simulink library "dragTurbine"  (R2020a)
settings: Solver=VariableStepAuto  StartTime=0.0  StopTime=10.0  RelTol=1e-3
undefined symbols (not defined in the file): alph, eta1, rho, tsrTab, vcl
libraries: simulink x3, vrlib x2, alphaBeta_ul x1, localApparentWind_ul x1
settings Model: Creator=Ayaz  LastModifiedBy=adabney
settings DataIOCC: ReturnWorkspaceOutputs=off
settings DebuggingCC: ArithmeticOperatorsInVariantConditions=warning
settings SFSimCC: CustomCodeUndefinedFunction=UseInterfaceOnly

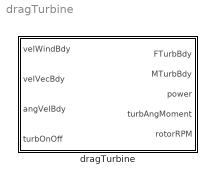
== system dragTurbine ==
  dragTurbine : Subsystem  TreatAsAtomicUnit=on  mask{vhcl=vcl}
      mask prompts: vhcl "Vehicle Object"

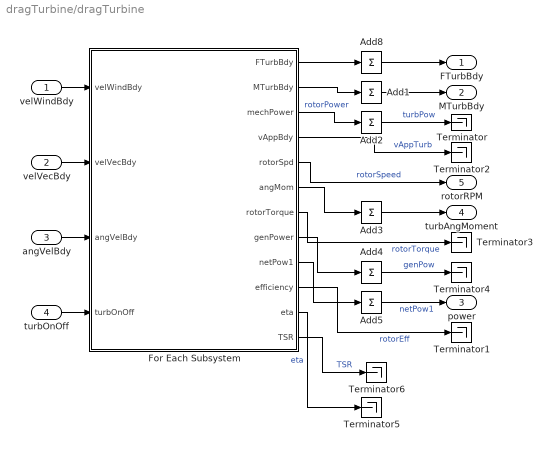
== system dragTurbine/dragTurbine ==
  velWindBdy : Inport
  velVecBdy : Inport  Port=2
  angVelBdy : Inport  Port=3
  turbOnOff : Inport  Port=4
  Add{1..3,8} (4 alike) : Sum  Inputs=1  CollapseMode=Specified dimension  CollapseDim=2
  Add4 : Sum  Inputs=1  CollapseDim=2
  Add5 : Sum  Inputs=1  CollapseDim=2
  For Each Subsystem : Subsystem  TreatAsAtomicUnit=on  mask{rho=rho, turb_struct=vhcl.struct('OCT.turb'), vhcl=vhcl}
      mask prompts: rho "Fluid Density"; turb_struct "Turbine Structure"; vhcl "Vehicle"
  Terminator{,1..6} (7 alike) : Terminator
  FTurbBdy : Outport  PortDimensions=[3,1]  VectorParamsAs1DForOutWhenUnconnected=off
  MTurbBdy : Outport  Port=2  PortDimensions=[3,1]  VectorParamsAs1DForOutWhenUnconnected=off
  power : Outport  Port=3  PortDimensions=[1,1]  VectorParamsAs1DForOutWhenUnconnected=off
  turbAngMoment : Outport  Port=4  PortDimensions=[3,1]  VectorParamsAs1DForOutWhenUnconnected=off
  rotorRPM : Outport  Port=5  VectorParamsAs1DForOutWhenUnconnected=off
  wires:
  velVecBdy/1 -> For Each Subsystem/2(velVecBdy)
  angVelBdy/1 -> For Each Subsystem/3(angVelBdy)
  turbOnOff/1 -> For Each Subsystem/4(turbOnOff)
  For Each Subsystem/1(FTurbBdy) -> Add8/1
  For Each Subsystem/2(MTurbBdy) -> Add1/1
  velWindBdy/1 -> For Each Subsystem/1(velWindBdy)
  Add8/1 -> FTurbBdy/1
  Add1/1 -> MTurbBdy/1
  For Each Subsystem/5(rotorSpd) -> rotorRPM/1  "rotorSpeed"
  For Each Subsystem/3(mechPower) -> Add2/1  "rotorPower"
  Add2/1 -> Terminator/1  "turbPow"
  For Each Subsystem/6(angMom) -> Add3/1
  Add3/1 -> turbAngMoment/1
  For Each Subsystem/4(vAppBdy) -> Terminator2/1  "vAppTurb"
  For Each Subsystem/7(rotorTorque) -> Terminator3/1  "rotorTorque"
  For Each Subsystem/8(genPower) -> Add4/1
  Add4/1 -> Terminator4/1  "genPow"
  For Each Subsystem/10(efficiency) -> Terminator1/1  "rotorEff"
  For Each Subsystem/9(netPow1) -> Add5/1
  Add5/1 -> power/1  "netPow1"
  For Each Subsystem/11(eta) -> Terminator5/1  "eta"
  For Each Subsystem/12(TSR) -> Terminator6/1  "TSR"

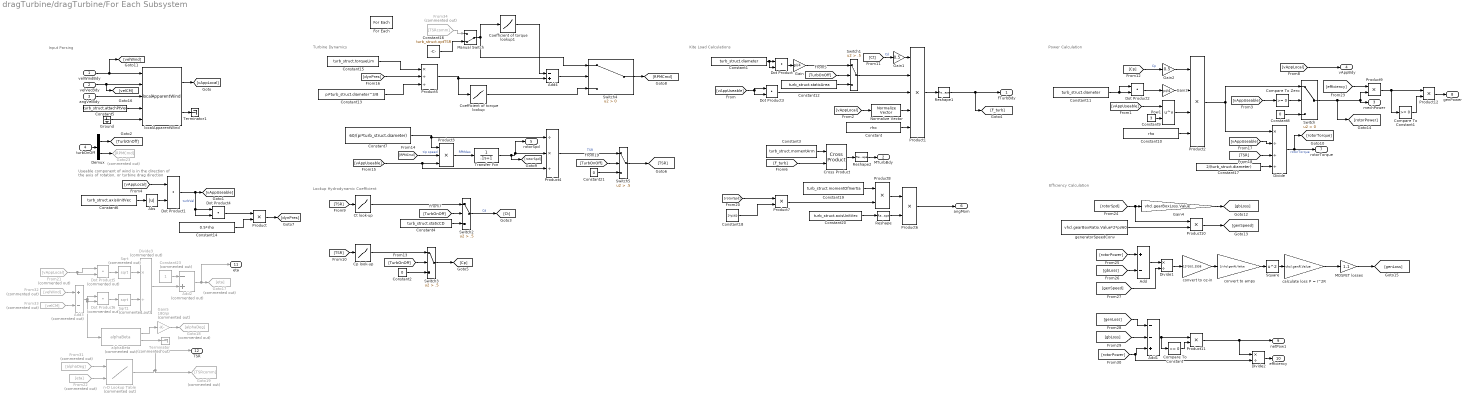
== system dragTurbine/dragTurbine/For Each Subsystem ==
  note: Lookup Hydrodynamic Coefficient
  note: Efficiency Calculation
  note: Input Parsing
  note: Turbine Dynamics
  note: Kite Load Calculations
  note: Power Calculation
  note: Useable component of wind is in the direction of
      | the axis of rotation, or turbine drag direction
  velWindBdy : Inport  Partition=on  PartitionDimension=2  PartitionWidth=1  PartitionOffset=0
  velVecBdy : Inport  Port=2
  angVelBdy : Inport  Port=3
  turbOnOff : Inport  Port=4
  Abs : Abs
  Add : Sum  Inputs=+-
  Add1 : Sum  Inputs=--+
  Add2 : Sum  Commented=on  Inputs=-+
  Add3 : Sum  Commented=on  Inputs=+-
  Add4 : Sum  Inputs=-+
  Coefficient of torque lookup : Lookup_n-D  NumberOfTableDimensions=1  BreakpointsForDimension1=turb_struct.tauCoefLookup  Table=turb_struct.tauCoefTSR  InternalRulePriority=Speed  RndMeth=Simplest  InputSameDT=on
  Coefficient of torque lookup1 : Lookup_n-D  NumberOfTableDimensions=1  BreakpointsForDimension1=turb_struct.tauCoefTSR(end:-1:1)  Table=turb_struct.tauCoefLookup(end:-1:1)  InternalRulePriority=Speed  RndMeth=Simplest  InputSameDT=on
  Compare To Constant : simulink/Logic and Bit Operations/Compare To Constant  relop=>=  const=0  OutDataTypeStr=boolean
  Compare To Constant1 : simulink/Logic and Bit Operations/Compare To Constant  relop=>=  const=0  OutDataTypeStr=boolean
  Compare To Zero : simulink/Logic and Bit Operations/Compare To Zero  relop=>=  OutDataTypeStr=boolean
  Constant : Constant  Value=rho
  Constant1 : Constant  Value=turb_struct.diameter  VectorParams1D=off
  Constant10 : Constant  Value=rho
  Constant11 : Constant  Value=turb_struct.diameter  VectorParams1D=off
  Constant12 : Constant  Value=turb_struct.staticArea  VectorParams1D=off
  Constant13 : Constant  Value=pi*turb_struct.diameter^3/8
  Constant14 : Constant  Value=0.5*rho
  Constant15 : Constant  Value=turb_struct.torqueLim
  Constant16 : Constant  Value=turb_struct.optTSR
  Constant17 : Constant  Value=2/(turb_struct.diameter)
  Constant18 : Constant  Value=2*pi/60
  Constant19 : Constant  Value=turb_struct.momentOfInertia
  Constant2 : Constant  Value=0
  Constant20 : Constant  Value=turb_struct.axisUnitVec
  Constant21 : Constant  Value=0
  Constant23 : Constant  Commented=on
  Constant3 : Constant  Value=turb_struct.momentArm
  Constant4 : Constant  Value=turb_struct.staticCD
  Constant5 : Constant  Value=turb_struct.attachPtVec
  Constant6 : Constant  Value=turb_struct.axisUnitVec
  Constant7 : Constant  Value=60/(pi*turb_struct.diameter)
  Constant8 : Constant  Value=0
  Constant9 : Constant  Value=3
  Cp look-up : Lookup_n-D  NumberOfTableDimensions=1  BreakpointsForDimension1=turb_struct.RPMref  Table=turb_struct.CpLookup  InternalRulePriority=Speed  RndMeth=Simplest  InputSameDT=on
  Cross Product : vrlib/Utilities/Cross Product
  Ct look-up : Lookup_n-D  NumberOfTableDimensions=1  BreakpointsForDimension1=turb_struct.RPMref  Table=turb_struct.CtLookup  InternalRulePriority=Speed  RndMeth=Simplest  InputSameDT=on
  Demux : Demux  Outputs=2
  Divide : Product  Inputs=*///
  Divide1 : Product  Inputs=*/
  Divide2 : Product  Inputs=*/
  Divide3 : Product  Commented=on  Inputs=*/
  Dot Product{,1..4} (5 alike) : DotProduct  InputSameDT=on  OutDataTypeStr=Inherit: Inherit via internal rule
  Dot Product5 : DotProduct  Commented=on  InputSameDT=on  OutDataTypeStr=Inherit: Inherit via internal rule
  Dot Product6 : DotProduct  Commented=on  InputSameDT=on  OutDataTypeStr=Inherit: Inherit via internal rule
  For Each : ForEach  DisableCoverage=on  IterateSubsysMaskParameter=off,on,off,on  SubsysMaskParameterIterationDimension=1,2,1,2
  From21 : From  Commented=on  GotoTag=vAppLocal
  From22 : From  Commented=on  GotoTag=eta
  From31 : From  Commented=on  GotoTag=alphaDeg
  From32 : From  Commented=on  GotoTag=velWind
  From33 : From  Commented=on  GotoTag=velCM
  From34 : From  Commented=on  GotoTag=TSRcomm
  Gain : Gain  Gain=pi/4
  Gain1 : Gain  Gain=0.5
  Gain2 : Gain  Gain=0.5
  Gain3 : Gain  Gain=pi/4
  Gain4 : Gain  Gain=vhcl.gearBoxLoss.Value
  Gain5 : Gain  Commented=on  Gain=180/pi
  Goto17 : Goto  Commented=on  GotoTag=eta
  Goto18 : Goto  Commented=on  GotoTag=alphaDeg
  Goto19 : Goto  Commented=on  GotoTag=TSRcomm
  Goto23 : Goto  Commented=on  GotoTag=RPMCmd
  Ground : Ground
  MOSFET losses : Gain  Gain=1.1
  Manual Switch : ManualSwitch  CurrentSetting=0
  Normalize Vector : vrlib/Utilities/Normalize Vector  maxzero=0
  Pow1 : Math  Operator=pow  SignedPower=on  RndMeth=Zero  SaturateOnIntegerOverflow=on
  Product{,6..12} (8 alike) : Product
  Product1 : Product  Inputs=5
  Product2 : Product  Inputs=4
  Product3 : Product  Inputs=3
  Product4 : Product  Inputs=/*/
  Product5 : Product  Inputs=*//
  Reshape : Reshape  OutputDimensionality=Column vector (2-D)
  Reshape1 : Reshape  OutputDimensionality=Column vector (2-D)
  Reshape2 : Reshape  OutputDimensionality=Column vector (2-D)
  Sqrt : Sqrt  Commented=on  SaturateOnIntegerOverflow=on
  Sqrt1 : Sqrt  Commented=on  SaturateOnIntegerOverflow=on
  Square : Math  Operator=square  SaturateOnIntegerOverflow=on
  Switch : Switch  Criteria=u2 > Threshold
  Switch{1..3,5} (4 alike) : Switch  Criteria=u2 > Threshold  Threshold=.5
  Switch4 : Switch  Criteria=u2 > Threshold
  Terminator : Terminator  Commented=on
  Terminator1 : Terminator
  Transfer Fcn : TransferFcn  Denominator=[.1 1]
  alphaBeta : alphaBeta_ul/alphaBeta  Commented=on  SystemSampleTime=-1  Latency=0  AutoFrameSizeCalculation=off
  calculate loss P = I^2R : Gain  Gain=vhcl.genR.Value
  convert to amps : Gain  Gain=1/vhcl.genKt.Value
  convert to oz-in : Gain  Gain=12*16/1.3558
  generatorSpeedConv : Constant  Value=vhcl.gearBoxRatio.Value*2*pi/60
  localApparentWind : localApparentWind_ul/localApparentWind  SystemSampleTime=-1  Latency=0  AutoFrameSizeCalculation=off
  n-D Lookup Table : Lookup_n-D  Commented=on  BreakpointsForDimension1=alph  BreakpointsForDimension2=eta1  BreakpointsForDimension3=[5, 7]  BreakpointsForDimension2FirstPoint=-.3  BreakpointsForDimension1Spacing=.1  BreakpointsForDimension2Spacing=.01  Table=tsrTab.tsr  InternalRulePriority=Speed  RndMeth=Simplest  InputSameDT=on
  FTurbBdy : Outport  PortDimensions=[3,1]  ConcatenationDimension=2  VectorParamsAs1DForOutWhenUnconnected=off
  MTurbBdy : Outport  Port=2  PortDimensions=[3,1]  ConcatenationDimension=2  VectorParamsAs1DForOutWhenUnconnected=off
  mechPower : Outport  Port=3  PortDimensions=[1,1]  ConcatenationDimension=2  VectorParamsAs1DForOutWhenUnconnected=off
  vAppBdy : Outport  Port=4  PortDimensions=[3,1]  ConcatenationDimension=2  VectorParamsAs1DForOutWhenUnconnected=off
  rotorSpd : Outport  Port=5  ConcatenationDimension=2
  angMom : Outport  Port=6  ConcatenationDimension=2
  rotorTorque : Outport  Port=7  ConcatenationDimension=1
  genPower : Outport  Port=8  ConcatenationDimension=1
  netPow1 : Outport  Port=9  ConcatenationDimension=1
  efficiency : Outport  Port=10  ConcatenationDimension=1
  eta : Outport  Port=11  ConcatenationDimension=1
  TSR : Outport  Port=12  ConcatenationDimension=1
  wires:
  Gain2/1 -> Product2/1
  angVelBdy/1 -> localApparentWind/3
  Constant11/1 -> Dot Product2/2, Dot Product2/1
  [vAppUseable] -> Dot Product3/1, Dot Product3/2
  [TSR] -> Ct look-up/1
  Constant10/1 -> Product2/4
  [vAppUseable] -> Pow1/1
  Dot Product2/1 -> Gain3/1
  [vAppLocal] -> Dot Product1/1
  Cp look-up/1 -> Switch3/1
  Gain3/1 -> Product2/2
  Dot Product/1 -> Gain/1
  [vAppUseable] -> Compare To Zero/1
  Cross Product/1 -> Reshape2/1
  Constant8/1 -> Switch/3
  Demux/1 -> [TurbOnOff]
  Switch/1 -> [rotorPower], mechPower/1, Product9/2
  Gain1/1 -> Product1/1
  Dot Product4/1 -> Product/1
  Gain/1 -> Switch1/1
  Pow1/1 -> Product2/3
  Constant9/1 -> Pow1/2
  Constant6/1 -> Abs/1
  Constant3/1 -> Cross Product/1
  Product3/1 -> Transfer Fcn/1  "RPMdes"
  Compare To Zero/1 -> Switch/2
  Reshape2/1 -> MTurbBdy/1
  Reshape1/1 -> FTurbBdy/1, [F_turb]
  localApparentWind/1 -> [vAppLocal]
  Constant5/1 -> localApparentWind/4
  [vAppLocal] -> vAppBdy/1
  turbOnOff/1 -> Demux/1
  localApparentWind/2 -> Terminator1/1
  [Cp] -> Gain2/1  "Cp"
  Constant2/1 -> Switch3/3
  Abs/1 -> Dot Product1/2
  [TurbOnOff] -> Switch3/2
  [TSR] -> Divide/3
  [vAppLocal] -> Normalize Vector/1
  [TSR] -> Cp look-up/1
  Constant1/1 -> Dot Product/1, Dot Product/2
  Switch3/1 -> [Cp]
  velVecBdy/1 -> [velCM], localApparentWind/2
  Normalize Vector/1 -> Product1/4
  [TurbOnOff] -> Switch2/2
  [Ct] -> Gain1/1  "Cd"
  Constant7/1 -> Product4/1, Product3/1
  [F_turb] -> Cross Product/2
  Product5/1 -> Coefficient of torque lookup/1, Add4/2
  [RPMCmd] -> Product3/2  "tip speed"
  Demux/2 -> Goto23/1
  Switch2/1 -> [Ct]  "Cd"
  Constant12/1 -> Switch1/3
  Constant15/1 -> Product5/1
  Constant14/1 -> Product/2
  [vAppUseable] -> Product3/3, Product4/3
  Constant/1 -> Product1/5
  Dot Product3/1 -> Product1/3
  Constant16/1 -> Manual Switch/2
  Product4/1 -> Switch5/1  "TSR"
  Constant13/1 -> Product5/3
  Constant4/1 -> Switch2/3
  Product/1 -> [dynPres]
  Coefficient of torque lookup/1 -> Switch4/3
  [dynPres] -> Product5/2
  Ct look-up/1 -> Switch2/1
  Ground/1 -> localApparentWind/5
  [vAppUseable] -> Divide/2
  Product1/1 -> Reshape1/1
  Switch4/1 -> [RPMCmd]
  Switch1/1 -> Product1/2
  Divide/1 -> [rotorTorque], rotorTorque/1  "rotorTorque"
  Product2/1 -> Switch/1, Divide/1
  Constant17/1 -> Divide/4
  Dot Product1/1 -> [vAppUseable], Dot Product4/1, Dot Product4/2  "turbVel"
  [TurbOnOff] -> Switch1/2
  Constant20/1 -> Reshape/1
  Reshape/1 -> Product6/2
  Constant19/1 -> Product8/1
  Product6/1 -> angMom/1
  Product7/1 -> Product8/2
  Product8/1 -> Product6/1
  [rotorSpd] -> Product7/1
  Constant18/1 -> Product7/2
  [TurbOnOff] -> Switch5/2
  Switch5/1 -> [TSR]
  Constant21/1 -> Switch5/3
  [efficiency] -> Product9/1
  Transfer Fcn/1 -> [rotorSpd], Product4/2, rotorSpd/1
  [rotorSpd] -> Product10/1, Gain4/1
  Gain4/1 -> [gbLoss]
  generatorSpeedConv/1 -> Product10/2
  Product10/1 -> [genSpeed]
  [gbLoss] -> Add/2
  [rotorPower] -> Add/1
  Add/1 -> Divide1/1
  [genSpeed] -> Divide1/2
  Divide1/1 -> convert to oz-in/1
  convert to oz-in/1 -> convert to amps/1
  convert to amps/1 -> Square/1
  Square/1 -> calculate loss P = I^2R/1
  calculate loss P = I^2R/1 -> MOSFET losses/1
  [gbLoss] -> Add1/2
  [genLoss] -> Add1/1
  [rotorPower] -> Divide2/2, Add1/3
  Product11/1 -> Divide2/1, netPow1/1
  Compare To Constant/1 -> Product11/2
  Add1/1 -> Compare To Constant/1, Product11/1
  Product12/1 -> genPower/1
  Compare To Constant1/1 -> Product12/2
  Product9/1 -> Product12/1, Compare To Constant1/1
  Divide2/1 -> efficiency/1
  MOSFET losses/1 -> [genLoss]
  Dot Product5/1 -> Sqrt/1
  From21/1 -> Dot Product5/2, Dot Product5/1
  velWindBdy/1 -> localApparentWind/1, [velWind]
  From33/1 -> Add3/2
  From32/1 -> Add3/1
  Dot Product6/1 -> Sqrt1/1
  Add3/1 -> Dot Product6/1, Dot Product6/2, alphaBeta/1
  Sqrt/1 -> Divide3/1
  Sqrt1/1 -> Divide3/2
  Divide3/1 -> Add2/2
  Constant23/1 -> Add2/1
  Add2/1 -> eta/1, Goto17/1
  alphaBeta/1 -> Gain5/1
  Gain5/1 -> Goto18/1
  alphaBeta/2 -> Terminator/1
  From22/1 -> n-D Lookup Table/2
  From31/1 -> n-D Lookup Table/1
  n-D Lookup Table/1 -> Goto19/1, TSR/1
  From34/1 -> Manual Switch/1
  Coefficient of torque lookup1/1 -> Add4/1
  Add4/1 -> Switch4/2
  Manual Switch/1 -> Coefficient of torque lookup1/1, Switch4/1
